simulink model "control_structure_b"  (R2015a)
settings: Solver=ode45  StartTime=0.0  StopTime=t_stop  MaxStep=0.01  MinStep=0.001  RelTol=1e-3
values from neighbouring files (symbols this model uses):
  A_dA = 0.3    [ex1.m]    (also in ex2.m = 0.01; ex3.m = 0)
  A_dT = 0    [ex1.m]    (also in ex2.m; ex3.m)
  A_dY = 0    [ex1.m]    (also in ex2.m = 0.1; ex3.m)
  A_r = 0.1    [ex1.m]    (also in ex2.m = 0; ex3.m = 3)
libraries: cstblocks x2
settings Model: Creator=Riccardo  LastModifiedBy=Riccardo

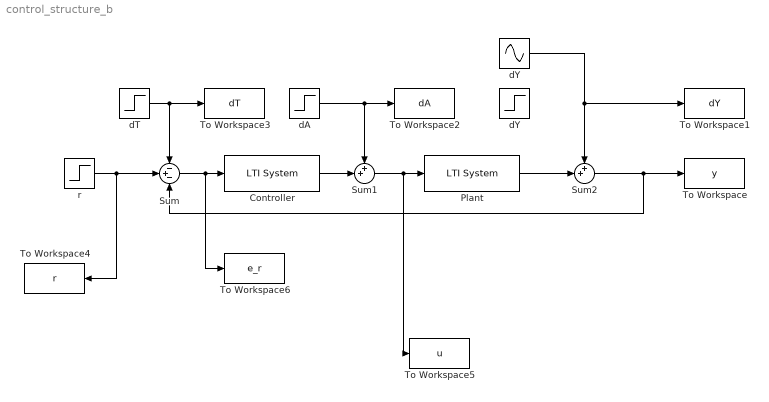
== system control_structure_b ==
  Controller : cstblocks/LTI System  sys=C  IC=[]
  Plant : cstblocks/LTI System  sys=G  IC=[]
  Sum : Sum  Inputs=-+-
  Sum1 : Sum  Inputs=++|
  Sum2 : Sum  Inputs=++|
  To Workspace : ToWorkspace  VariableName=y  SaveFormat=Structure With Time  SampleTime=-1
  To Workspace1 : ToWorkspace  VariableName=dY  SaveFormat=Structure With Time  SampleTime=-1
  To Workspace2 : ToWorkspace  VariableName=dA  SaveFormat=Structure With Time  SampleTime=-1
  To Workspace3 : ToWorkspace  VariableName=dT  SaveFormat=Structure With Time  SampleTime=-1
  To Workspace4 : ToWorkspace  VariableName=r  SaveFormat=Structure With Time  SampleTime=-1
  To Workspace5 : ToWorkspace  VariableName=u  SaveFormat=Structure With Time  SampleTime=-1
  To Workspace6 : ToWorkspace  VariableName=e_r  SaveFormat=Structure With Time  SampleTime=-1
  "dA " : Step  Time=0  After=A_dA  SampleTime=0
  "dT " : Step  Time=0  After=A_dT  SampleTime=0
  dY : Step  Time=0  After=A_dY  SampleTime=0
  "dY " : Sin  Amplitude=A_dY  Frequency=0.05  SampleTime=0
  "r " : Step  Time=0  After=A_r  SampleTime=0
  wires:
  "dT "/1 -> To Workspace3/1, Sum/1
  Sum/1 -> To Workspace6/1, Controller/1
  "dA "/1 -> To Workspace2/1, Sum1/1
  Sum1/1 -> To Workspace5/1, Plant/1
  Controller/1 -> Sum1/2
  Plant/1 -> Sum2/2
  Sum2/1 -> To Workspace/1, Sum/3
  "r "/1 -> To Workspace4/1, Sum/2
  "dY "/1 -> Sum2/1, To Workspace1/1
